simulink model "open_150W"  (R2024a)
settings: Solver=VariableStepAuto  StartTime=0.0  StopTime=0.5  RelTol=1e-3
libraries: spsCurrentMeasurementLib x4, spsSeriesRLCBranchLib x4, spsDiodeLib x2, spsIGBTDiodeLib x2, spsVoltageMeasurementLib x2, spsDCVoltageSourceLib x1, spsSawtoothGeneratorLib x1, sps_lib x1
settings Model: Creator=prana  LastModifiedBy=deepa

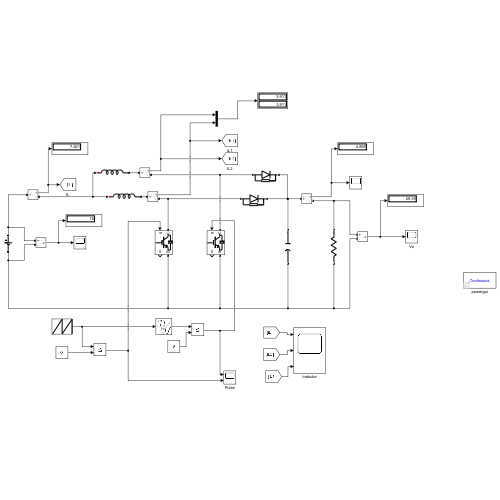
[thumbnail: Simulink's stored preview of the top-level diagram]
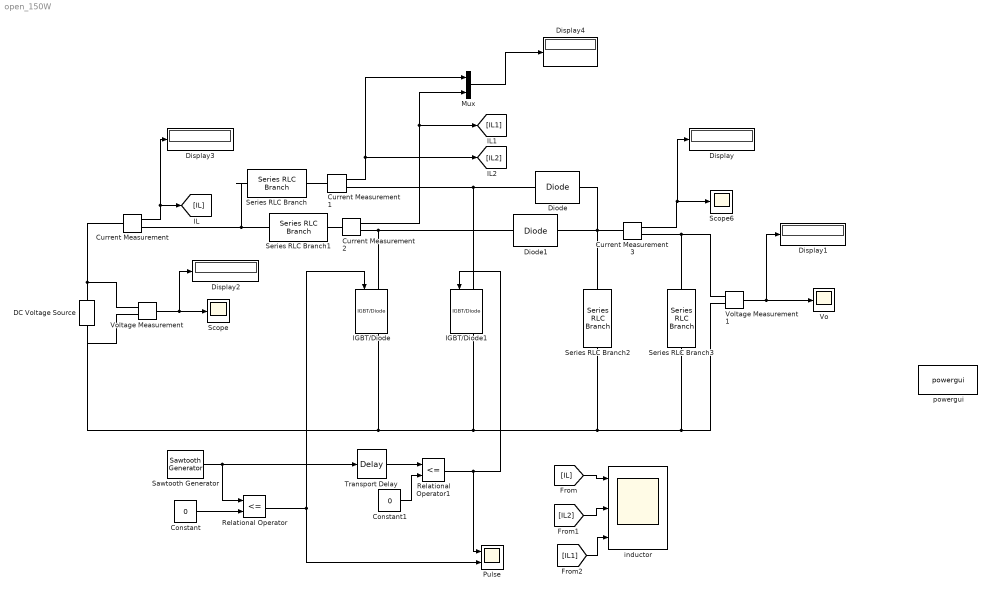
== system open_150W ==
  Constant : Constant  Value=0
  Constant1 : Constant  Value=0
  Current Measurement{,1..3} (4 alike) : spsCurrentMeasurementLib/Current Measurement  PhasorSimulation=off  OutputType=Complex  PSBequivalent=0
  DC Voltage Source : spsDCVoltageSourceLib/DC Voltage Source  Amplitude=15  Measurements=None
  Diode : spsDiodeLib/Diode  Ron=0.001  Lon=0  Vf=0.8  IC=0  UseSnubber=0  Rs=500  Cs=250e-9  Measurements=off
  Diode1 : spsDiodeLib/Diode  Ron=0.001  Lon=0  Vf=0.8  IC=0  UseSnubber=0  Rs=500  Cs=250e-9  Measurements=off
  Display{,1..4} (5 alike) : Display
  IGBT/Diode : spsIGBTDiodeLib/IGBT//Diode  Ron=1e-3  Rs=1e5  Cs=inf  Measurements=on
  IGBT/Diode1 : spsIGBTDiodeLib/IGBT//Diode  Ron=1e-3  Rs=1e5  Cs=inf  Measurements=on
  Mux : Mux  Inputs=2
  Pulse : Scope  NumInputPorts=2
      settings: Description=O/P V
  Relational Operator : RelationalOperator  Operator=<=  OutDataTypeStr=boolean  RndMeth=Simplest  InputSameDT=off
  Relational Operator1 : RelationalOperator  Operator=<=  OutDataTypeStr=boolean  RndMeth=Simplest  InputSameDT=off
  Sawtooth Generator : spsSawtoothGeneratorLib/Sawtooth Generator  Freq=10e3  Phase=0  Ts=0
  Scope : Scope
  Scope6 : Scope
  Series RLC Branch : spsSeriesRLCBranchLib/Series RLC Branch  LConnTagsString=__new0  RConnTagsString=__new0  BranchType=L  Resistance=1  Inductance=3.75e-4  SetiL0=off  InitialCurrent=0  Capacitance=1e-6  Setx0=off  InitialVoltage=0  Measurements=None
  Series RLC Branch1 : spsSeriesRLCBranchLib/Series RLC Branch  LConnTagsString=__new0  RConnTagsString=__new0  BranchType=L  Resistance=1  Inductance=3.75e-4  SetiL0=off  InitialCurrent=0  Capacitance=1e-6  Setx0=off  InitialVoltage=0  Measurements=None
  Series RLC Branch2 : spsSeriesRLCBranchLib/Series RLC Branch  LConnTagsString=__new0  RConnTagsString=__new0  BranchType=C  Resistance=1  Inductance=1e-3  SetiL0=off  InitialCurrent=0  Capacitance=8.33e-4  Setx0=off  InitialVoltage=0  Measurements=None
  Series RLC Branch3 : spsSeriesRLCBranchLib/Series RLC Branch  LConnTagsString=__new0  RConnTagsString=__new0  BranchType=R  Resistance=6  Inductance=1e-3  SetiL0=off  InitialCurrent=0  Capacitance=1e-6  Setx0=off  InitialVoltage=0  Measurements=None
  Transport Delay : TransportDelay  DelayTime=2e-4
  Vo : Scope
      settings: Description=O/P V
  Voltage Measurement : spsVoltageMeasurementLib/Voltage Measurement  PhasorSimulation=off  OutputType=Complex  PSBequivalent=0
  Voltage Measurement1 : spsVoltageMeasurementLib/Voltage Measurement  PhasorSimulation=off  OutputType=Complex  PSBequivalent=0
  inductor : Scope  NumInputPorts=3
      settings: Description=O/P V
  powergui : sps_lib/powergui  Priority=1  SimulationMode=Continuous  SampleTime=50e-6  frequency=60  Iterations=50  frequencyindice=0  Pbase=100e6  ErrMax=1e-4  UnitsV=kV  UnitsW=MW  buscounter=0  FunctionMessages=off  echomessages=off  EnableUseOfTLC=off  CurrentSourceSwitches=off  DisableSnubberDevices=off  DisableRonSwitches=off  DisableVfSwitches=off  DisplayEquations=off  AutomaticDiscreteSolvers=off  SolverType=Tustin/Backward Euler (TBE)  Interpol=off  ExternalGateDelay=off  methode=off  Ts=100  x0status=blocks  SPID=on  SwTol=0  HookPort=off  NonlinearTolerance=1e-4  nMaxIteration=100  ContinueOnMaxIteration=off  RestoreLinks=warning  ResistiveCurrentMeasurement=off  Frange=[0:2:500]  Ylog=off  Xlog=on  ShowGrid=off  save=off  variable=ZData  structure=0  ZoomFFT=off  StartTime=0.0  cycles=1  DisplayStyle=1  fundamental=60  FreqAxis=off  MaxFrequency=1000  frequencyindicesteady=1  RmsSteady=1  display=off
  wires:
  Voltage Measurement/1 -> Display2/1, Scope/1
  Current Measurement/1 -> [IL], Display3/1
  Voltage Measurement1/1 -> Display1/1, Vo/1
  Current Measurement1/1 -> Mux/1, [IL2]
  Current Measurement2/1 -> [IL1], Mux/2
  Current Measurement3/1 -> Display/1, Scope6/1
  Relational Operator/1 -> Pulse/2, IGBT/Diode/1
  Mux/1 -> Display4/1
  Sawtooth Generator/1 -> Transport Delay/1, Relational Operator/1
  Constant/1 -> Relational Operator/2
  Transport Delay/1 -> Relational Operator1/1
  Constant1/1 -> Relational Operator1/2
  Relational Operator1/1 -> Pulse/1, IGBT/Diode1/1
  [IL] -> inductor/1
  [IL2] -> inductor/2
  [IL1] -> inductor/3
  connections:
  Voltage Measurement/LConn1 -- DC Voltage Source/RConn1 -- Current Measurement/LConn1
  Series RLC Branch1/LConn1 -- Series RLC Branch/LConn1 -- Current Measurement/RConn1
  Current Measurement1/LConn1 -- Series RLC Branch/RConn1
  Current Measurement2/LConn1 -- Series RLC Branch1/RConn1
  Diode/LConn1 -- IGBT/Diode1/LConn1 -- Current Measurement1/RConn1
  Diode1/LConn1 -- IGBT/Diode/LConn1 -- Current Measurement2/RConn1
  Current Measurement3/LConn1 -- Series RLC Branch2/LConn1 -- Diode1/RConn1 -- Diode/RConn1
  Current Measurement3/RConn1 -- Series RLC Branch3/LConn1 -- Voltage Measurement1/LConn1
  Voltage Measurement1/LConn2 -- Series RLC Branch2/RConn1 -- IGBT/Diode1/RConn1 -- IGBT/Diode/RConn1 -- Voltage Measurement/LConn2 -- DC Voltage Source/LConn1 -- Series RLC Branch3/RConn1
